simulink model "battery_model"  (R2016a)
settings: Solver=ode23tb  StartTime=0.0  StopTime=60  RelTol=1e-3
values from neighbouring files (symbols this model uses):
  Cnom = 5    [battery_parameters.m]
  etaC = 0.93    [battery_parameters.m]
  Mp = 2    [battery_parameters.m]
  Ns = 100    [battery_parameters.m]
  R1 = 10e-3    (= 0.01)    [battery_parameters.m]
  Rn = 10e-3    (= 0.01)    [battery_parameters.m]
  Rp = 10e-3    (= 0.01)    [battery_parameters.m]
  SOC_0 = 0.5    [battery_parameters.m]
  tau1 = 100    [battery_parameters.m]
  tauh = 50    [battery_parameters.m]
  Vm = 20e-3    (= 0.02)    [battery_parameters.m]
undefined symbols (not defined in the file or in its folder): V_soc
libraries: simulink x1
settings Model: Creator=Gorkem  LastModifiedBy=Gorkem

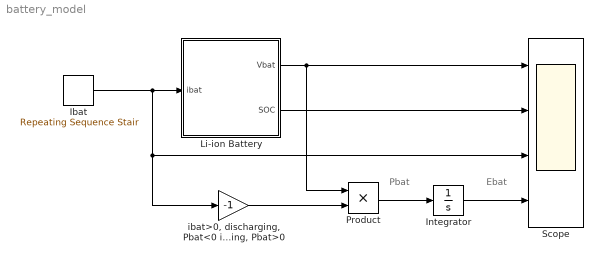
== system battery_model ==
  note: Ebat
  note: Pbat
  Ibat : simulink/Sources/Repeating Sequence Stair  OutValues=[-10 0 -10 0 10 0 10 0 -10]  tsamp=7.5  OutMin=[]  OutMax=[]  OutDataTypeStr=double  OutputDataTypeScalingMode=double  OutDataType=fixdt(0,8)  ConRadixGroup=Best Precision: Vector-wise  OutScaling=2^-12
  Integrator : Integrator
  Li-ion Battery : Subsystem
  Product : Product
  Scope : Scope  NumInputPorts=4
  "ibat>0, discharging, Pbat<0 ibat<0, charging, Pbat>0" : Gain  Gain=-1
  wires:
  Li-ion Battery/1(Vbat) -> Product/1, Scope/1
  Li-ion Battery/2(SOC) -> Scope/2
  Ibat/1 -> "ibat>0, discharging, Pbat<0 ibat<0, charging, Pbat>0"/1, Scope/3, Li-ion Battery/1(ibat)
  Product/1 -> Integrator/1
  "ibat>0, discharging, Pbat<0 ibat<0, charging, Pbat>0"/1 -> Product/2
  Integrator/1 -> Scope/4

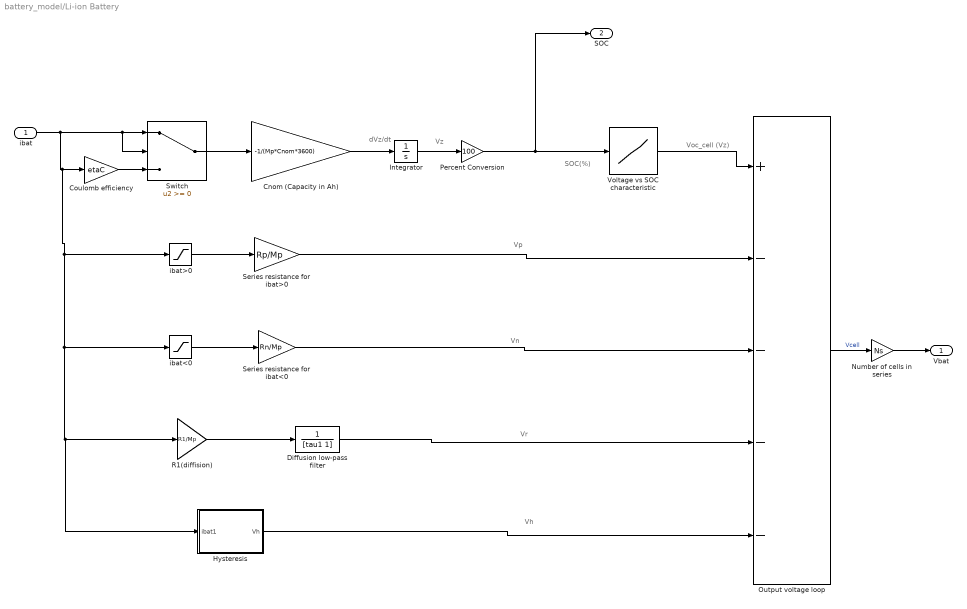
== system battery_model/Li-ion Battery ==
  note: Voc_cell (Vz)
  note: SOC(%)
  note: Vz
  note: Vh
  note: Vr
  note: Vn
  note: Vp
  note: dVz/dt
  ibat : Inport
  Cnom (Capacity in Ah) : Gain  Gain=-1/(Mp*Cnom*3600)
  Coulomb efficiency : Gain  Gain=etaC
  Diffusion low-pass filter : TransferFcn  Denominator=[tau1 1]
  Hysteresis : Subsystem
  Integrator : Integrator  InitialCondition=SOC_0  LimitOutput=on  UpperSaturationLimit=1  LowerSaturationLimit=0
  Number of cells in series : Gain  Gain=Ns
  Output voltage loop : Sum  Inputs=+----
  "Percent Conversion " : Gain  Gain=100
  R1(diffision) : Gain  Gain=R1/Mp
  Series resistance for ibat<0 : Gain  Gain=Rn/Mp
  Series resistance for ibat>0 : Gain  Gain=Rp/Mp
  Switch : Switch
  Voltage vs SOC characteristic : Lookup_n-D  NumberOfTableDimensions=1  BreakpointsForDimension1=[0:9900]/100  Table=V_soc  InternalRulePriority=Speed  RndMeth=Simplest  InputSameDT=on
  ibat<0 : Saturate  UpperLimit=0  LowerLimit=-inf
  ibat>0 : Saturate  UpperLimit=inf  LowerLimit=0
  Vbat : Outport
  SOC : Outport  Port=2
  wires:
  R1(diffision)/1 -> Diffusion low-pass filter/1
  Diffusion low-pass filter/1 -> Output voltage loop/4
  Series resistance for ibat>0/1 -> Output voltage loop/2
  Integrator/1 -> "Percent Conversion "/1
  "Percent Conversion "/1 -> SOC/1, Voltage vs SOC characteristic/1
  Series resistance for ibat<0/1 -> Output voltage loop/3
  Hysteresis/1(Vh) -> Output voltage loop/5
  ibat/1 -> Hysteresis/1(ibat1), R1(diffision)/1, ibat<0/1, ibat>0/1, Coulomb efficiency/1, Switch/2, Switch/1
  Number of cells in series/1 -> Vbat/1
  Output voltage loop/1 -> Number of cells in series/1  "Vcell"
  Voltage vs SOC characteristic/1 -> Output voltage loop/1
  ibat>0/1 -> Series resistance for ibat>0/1
  Coulomb efficiency/1 -> Switch/3
  Switch/1 -> Cnom (Capacity in Ah)/1
  Cnom (Capacity in Ah)/1 -> Integrator/1
  ibat<0/1 -> Series resistance for ibat<0/1

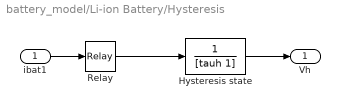
== system battery_model/Li-ion Battery/Hysteresis ==
  ibat1 : Inport
  Hysteresis state : TransferFcn  Denominator=[tauh 1]
  Relay : Relay  OnSwitchValue=0.01  OffSwitchValue=-0.01  OnOutputValue=Vm  OffOutputValue=-Vm
  Vh : Outport
  wires:
  Relay/1 -> Hysteresis state/1
  ibat1/1 -> Relay/1
  Hysteresis state/1 -> Vh/1
